simulink model "CONTROL_TESTING"  (R2024a)
settings: Solver=VariableStepAuto  StartTime=0.0  StopTime=inf  RelTol=1e-3
values from neighbouring files (symbols this model uses):
  C = 0    [CONTROL_TESTING_VARIABLES.m]
  Direction_Pin = 0    [CONTROL_TESTING_VARIABLES.m]
  EN_Pin = 1    [CONTROL_TESTING_VARIABLES.m]
  FP_New_Max_Angle = 360    [CONTROL_TESTING_VARIABLES.m]
  FP_New_Max_Percent = 255    [CONTROL_TESTING_VARIABLES.m]
  FP_New_Min_Angle = 0    [CONTROL_TESTING_VARIABLES.m]
  FP_New_Min_Percent = 0    [CONTROL_TESTING_VARIABLES.m]
  FP_Old_Max = 5    [CONTROL_TESTING_VARIABLES.m]
  FP_Old_Min = 0    [CONTROL_TESTING_VARIABLES.m]
  TB_New_Max_Angle = 360    [CONTROL_TESTING_VARIABLES.m]
  TB_New_Max_Percent = 255    [CONTROL_TESTING_VARIABLES.m]
  TB_New_Min_Angle = 0    [CONTROL_TESTING_VARIABLES.m]
  TB_New_Min_Percent = 0    [CONTROL_TESTING_VARIABLES.m]
  TB_Old_Max = 5    [CONTROL_TESTING_VARIABLES.m]
  TB_Old_Min = 0    [CONTROL_TESTING_VARIABLES.m]
libraries: fl_lib x11, nesl_utility x9, arduinolib x4, ee_lib x3, sdl_lib x1
(part 2 of 2)

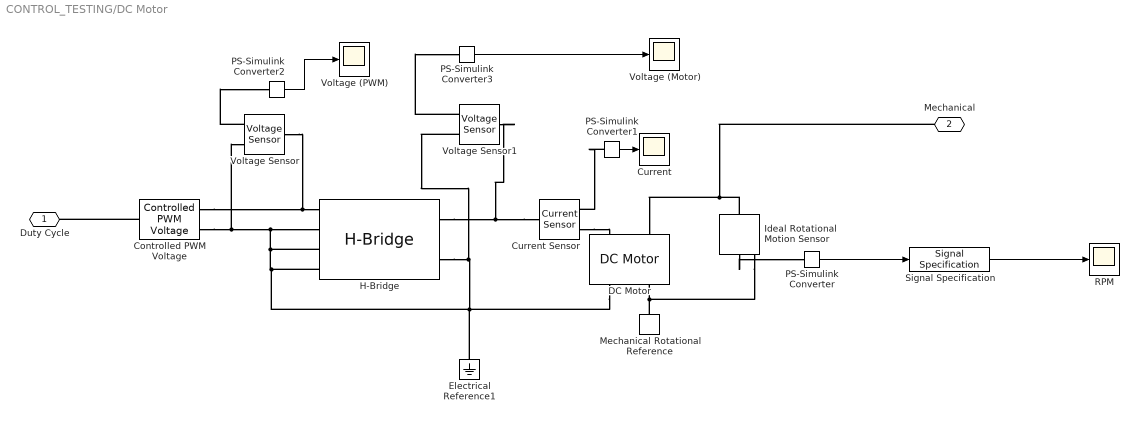
== system CONTROL_TESTING/DC Motor ==
  Controlled PWM Voltage : ee_lib/Integrated Circuits/Controlled PWM Voltage  F=2000 Hz  TD=0 s  pulse_width_offset=0 s  pulse_min=0 s  pwm_or_av=ee.enum.pwm_or_av.averaged  event_type=1  sample_time=1e-6 s  Vmin=0 V  Vmax=5 V  Vm=5 V  u_min=0  u_max=255
      settings: InternalSimscapePortConfiguration="{\"Bottom\":[],\"Left\":[{\"id\":\"u\",\"label\":\"u\",\"type\":\"input\"}],\"Right\":[{\"id\":\"p2\",\"label\":\"PWM\",\"type\":\"foundation.electrical.electrical\"},{\"id\":\"n2\",\"label\":\"REF\",\"type\":\"foundation.electrical.electrical\"}],\"Top\":[]}"
  Current : Scope
  Current Sensor : fl_lib/Electrical/Electrical Sensors/Current Sensor
  DC Motor : ee_lib/Electromechanical/Brushed Motors/DC Motor  field_option=ee.enum.field_option.pm  Rf=100 Ohm  Lf=1 H  Laf=0.15 H  If0=0 A  parameterization=ee.enum.dcparam_option.load_speed  Ra=3.9 Ohm  La=0.01 H  emf_or_torque=ee.enum.emf_or_torque.kv  Kv=0.072e-3 V/rpm  Ki=6.876e-4 N*m/A  T_stall=0.24e-3 N*m  w_max=4000 rpm  w_rated=2500 rpm  P_rated=10 W  V_rated=12 V  lam_param=ee.enum.lam_param.damping  i_noload=0 A  V_i_noload=1.5 V  J=0.0002 kg*m^2  lam=0.5e-5 N*m/(rad/s)  speed0=0 rpm  enable_fault_armature=simscape.enum.onoff.off  rev_faulted=1 / 3  G_faulted_armature=1e-5 S  fault_trigger_armature=ee.enum.faults.faultTrigger.temporal  t_fault_armature=1 s  max_permissible_current_armature=inf A  t_fail_on_current_armature=1 s  enable_fault_field=simscape.enum.onoff.off  G_faulted_field=1e-5 S  fault_trigger_field=ee.enum.faults.faultTrigger.temporal  t_fault_field=1 s  max_permissible_current_field=inf A  t_fail_on_current_field=1 s  fault_action=simscape.enum.assert.action.none  alpha=3.93e-3 1/K  Tmeas=25 degC  thermal_mass=100 J/K  initial_temperature=25 degC
      settings: LogSimulationData=on
  Electrical Reference1 : fl_lib/Electrical/Electrical Elements/Electrical Reference
  H-Bridge : ee_lib/Semiconductors & Converters/Converters/H-Bridge  supply_ports=ee.enum.supply_ports.hidesupply  pwm_or_av=ee.enum.pwm_or_av.averaged  regenerative_braking_mode=ee.enum.converters.regenerative_braking_mode.depends_on_rev  discontinuous=ee.enum.current_profile.continuous  freewheeling_mode=ee.enum.converters.freewheeling_mode.one_switch_one_diode  Rload=10 Ohm  Lload=1e-5 H  F=10 kHz  Venable=0.1 V  Vmax=5 V  Vreverse=2.5 V  Vbrake=0.1 V  Vm=12 V  Ron=0.1 Ohm  Don=0.05 Ohm  Goff=1e-6 S  Tmeas=298.15 K  Ron2=0.1 Ohm  Don2=0.05 Ohm  Tmeas2=398.15 K  thermal_mass=100 J/K  initial_temperature=298.15 K
  Ideal Rotational Motion Sensor : fl_lib/Mechanical/Mechanical Sensors/Ideal Rotational Motion Sensor  reference=foundation.enum.MeasurementReference.difference  acceleration_port=false  velocity_port=true  position_port=true  wrap_angle=simscape.enum.onoff.off  offset=0 rad
  Mechanical Rotational Reference : fl_lib/Mechanical/Rotational Elements/Mechanical Rotational Reference
  PS-Simulink Converter{,1..3} (4 alike) : nesl_utility/PS-Simulink Converter  PhysicalDomain=network_engine_domain  SubClassName=ps_output  LeftPortType=input  RightPortType=output  PseudoPeriodic=off  Frequencies=[]  VectorFormat=inherit  Unit=inherit  AffineConversion=off
  RPM : Scope
  Signal Specification : SignalSpecification  Unit=rpm
  Voltage (Motor) : Scope
  Voltage (PWM) : Scope
      settings: Priority=3
  Voltage Sensor : fl_lib/Electrical/Electrical Sensors/Voltage Sensor
  Voltage Sensor1 : fl_lib/Electrical/Electrical Sensors/Voltage Sensor
  Duty Cycle : PMIOPort  Side=Left
  Mechanical : PMIOPort  Port=2  Side=Right
  wires:
  PS-Simulink Converter1/1 -> Current/1
  PS-Simulink Converter/1 -> Signal Specification/1
  PS-Simulink Converter3/1 -> Voltage (Motor)/1
  PS-Simulink Converter2/1 -> Voltage (PWM)/1
  Signal Specification/1 -> RPM/1
  connections:
  H-Bridge/LConn4 -- Electrical Reference1/LConn1 -- Voltage Sensor1/RConn2 -- H-Bridge/RConn2 -- DC Motor/RConn1 -- H-Bridge/LConn3 -- Controlled PWM Voltage/RConn2 -- Voltage Sensor/RConn2 -- H-Bridge/LConn2
  H-Bridge/LConn1 -- Controlled PWM Voltage/RConn1 -- Voltage Sensor/LConn1
  PS-Simulink Converter1/LConn1 -- Current Sensor/RConn1
  Ideal Rotational Motion Sensor/LConn1 -- Mechanical/RConn1 -- DC Motor/LConn2
  Current Sensor/LConn1 -- Voltage Sensor1/LConn1 -- H-Bridge/RConn1
  Voltage Sensor1/RConn1 -- PS-Simulink Converter3/LConn1
  Ideal Rotational Motion Sensor/RConn1 -- Mechanical Rotational Reference/LConn1 -- DC Motor/RConn2
  Current Sensor/RConn2 -- DC Motor/LConn1
  Voltage Sensor/RConn1 -- PS-Simulink Converter2/LConn1
  Ideal Rotational Motion Sensor/RConn2 -- PS-Simulink Converter/LConn1
  Controlled PWM Voltage/LConn1 -- Duty Cycle/RConn1

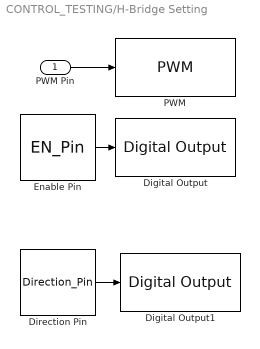
== system CONTROL_TESTING/H-Bridge Setting ==
  PWM Pin : Inport
  Digital Output : arduinolib/Digital Output  pinNumber=9  Direction=output  blockPlatform=arduino
  Digital Output1 : arduinolib/Digital Output  pinNumber=10  Direction=output  blockPlatform=arduino
  Direction Pin : Constant  Value=Direction_Pin
  Enable Pin : Constant  Value=EN_Pin
  PWM : arduinolib/PWM  pinNumber=5  frequencyType=Default  desiredFrequency=490.2  achievableFrequency=490.2
  wires:
  PWM Pin/1 -> PWM/1
  Enable Pin/1 -> Digital Output/1
  Direction Pin/1 -> Digital Output1/1

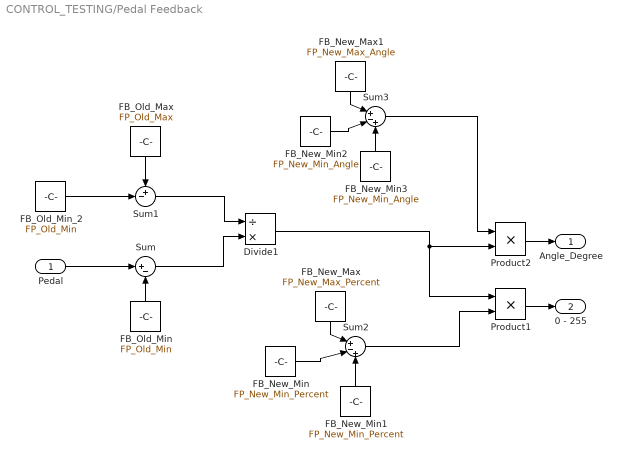
== system CONTROL_TESTING/Pedal Feedback ==
  Pedal : Inport
  Divide1 : Product  Inputs=/*
  FB_New_Max : Constant  Value=FP_New_Max_Percent
  FB_New_Max1 : Constant  Value=FP_New_Max_Angle
  FB_New_Min : Constant  Value=FP_New_Min_Percent
  FB_New_Min1 : Constant  Value=FP_New_Min_Percent
  FB_New_Min2 : Constant  Value=FP_New_Min_Angle
  FB_New_Min3 : Constant  Value=FP_New_Min_Angle
  FB_Old_Max : Constant  Value=FP_Old_Max
  FB_Old_Min : Constant  Value=FP_Old_Min
  FB_Old_Min_2 : Constant  Value=FP_Old_Min
  Product1 : Product
  Product2 : Product
  Sum : Sum  Inputs=|+-
  Sum1 : Sum  Inputs=+-|
  Sum2 : Sum  Inputs=|+-+
  Sum3 : Sum  Inputs=|+-+
  Angle_Degree : Outport
  0 - 255 : Outport  Port=2
  wires:
  FB_New_Min1/1 -> Sum2/3
  Product1/1 -> 0 - 255/1
  Divide1/1 -> Product1/1, Product2/2
  Sum2/1 -> Product1/2
  FB_New_Min2/1 -> Sum3/2
  FB_New_Max1/1 -> Sum3/1
  FB_New_Min/1 -> Sum2/2
  Sum3/1 -> Product2/1
  Sum/1 -> Divide1/2
  FB_Old_Min/1 -> Sum/2
  FB_New_Min3/1 -> Sum3/3
  FB_New_Max/1 -> Sum2/1
  FB_Old_Min_2/1 -> Sum1/2
  Sum1/1 -> Divide1/1
  Product2/1 -> Angle_Degree/1
  FB_Old_Max/1 -> Sum1/1
  Pedal/1 -> Sum/1

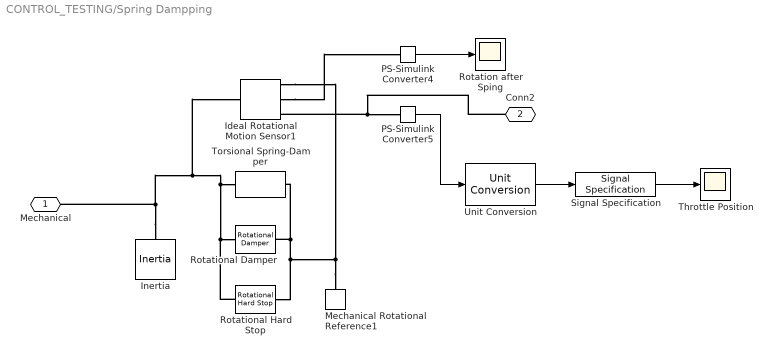
== system CONTROL_TESTING/Spring Dampping ==
  Ideal Rotational Motion Sensor1 : fl_lib/Mechanical/Mechanical Sensors/Ideal Rotational Motion Sensor  reference=foundation.enum.MeasurementReference.difference  acceleration_port=false  velocity_port=true  position_port=true  wrap_angle=true  offset=0 deg
  Inertia : fl_lib/Mechanical/Rotational Elements/Inertia  inertia=0.00000000001 kg*m^2  num_ports=foundation.enum.numPorts2.one  w_specify=off  w_priority=High  w=0 rad/s  w_nominal_specify=off  w_nominal_value=1  w_nominal_unit=rad/s  t_specify=off  t_priority=None  t=0 N*m  t_nominal_specify=off  t_nominal_value=1  t_nominal_unit=N*m
  Mechanical Rotational Reference1 : fl_lib/Mechanical/Rotational Elements/Mechanical Rotational Reference
  PS-Simulink Converter4 : nesl_utility/PS-Simulink Converter  PhysicalDomain=network_engine_domain  SubClassName=ps_output  LeftPortType=input  RightPortType=output  PseudoPeriodic=off  Frequencies=[]  VectorFormat=inherit  Unit=inherit  AffineConversion=off
  PS-Simulink Converter5 : nesl_utility/PS-Simulink Converter  PhysicalDomain=network_engine_domain  SubClassName=ps_output  LeftPortType=input  RightPortType=output  PseudoPeriodic=off  Frequencies=[]  VectorFormat=inherit  Unit=inherit  AffineConversion=off
  Rotation after Sping : Scope
  Rotational Damper : fl_lib/Mechanical/Rotational Elements/Rotational Damper  D=0.00001 N*m*s/rad  w_specify=off  w_priority=None  w=0 rad/s  w_nominal_specify=off  w_nominal_value=1  w_nominal_unit=rad/s  t_specify=off  t_priority=None  t=0 N*m  t_nominal_specify=off  t_nominal_value=1  t_nominal_unit=N*m
  Rotational Hard Stop : fl_lib/Mechanical/Rotational Elements/Rotational Hard Stop  upper_bnd=27.73873597 rad  lower_bnd=0 rad  model=simscape.enum.hardstop.smooth  stiff_up=1e6 N*m/rad  stiff_low=1e6 N*m/rad  D_up=0.1 N*m*s/rad  D_low=0.1 N*m*s/rad  transition=0.001 rad  coeff_rest=0.7  w_tol=0.1 rad/s  trq_tol=0.001 N*m  w_specify=off  w_priority=None  w=0 rad/s  w_nominal_specify=off  w_nominal_value=1  w_nominal_unit=rad/s  t_specify=off  t_priority=None  t=0 N*m  t_nominal_specify=off  t_nominal_value=1  t_nominal_unit=N*m  phi_specify=off  phi_priority=High  phi=0 rad  phi_nominal_specify=off  phi_nominal_value=1  phi_nominal_unit=rad  M_specify=off  M_priority=None  M=0
  Signal Specification : SignalSpecification  Unit=deg
  Throttle Position : Scope
  Torsional Spring-Damper : sdl_lib/Couplings & Drives/Torsional Spring-Damper  k=0.0020928 N*m/rad  mu_visc=0 N*m*s/rad  trq_coulomb=0 N*m  static_kinetic_ratio=10  w_tol=0.001 rad/s  model_hardstop=sdl.enum.hardStopOffOn.off  upper_bound=10 deg  lower_bound=-10 deg  hardstop_model=simscape.enum.hardstop.smooth  k_endstop=1e6 N*m/rad  D_endstop=10 N*m*s/rad  transition=0.001 rad  coeff_rest=0.7  w_tol_hardstop=0.1 rad/s  trq_tol=0.001 N*m  x0=0 deg
      settings: InternalSimscapePortConfiguration="{\"Bottom\":[],\"Left\":[{\"id\":\"R\",\"label\":\"R\",\"type\":\"foundation.mechanical.rotational.rotational\"}],\"Right\":[{\"id\":\"C\",\"label\":\"C\",\"type\":\"foundation.mechanical.rotational.rotational\"}],\"Top\":[]}"
  Unit Conversion : UnitConversion
  Mechanical : PMIOPort  Side=Left
  Conn2 : PMIOPort  Port=2  Side=Right
  wires:
  PS-Simulink Converter4/1 -> Rotation after Sping/1
  Signal Specification/1 -> Throttle Position/1
  PS-Simulink Converter5/1 -> Unit Conversion/1
  Unit Conversion/1 -> Signal Specification/1
  connections:
  Ideal Rotational Motion Sensor1/RConn2 -- PS-Simulink Converter4/LConn1
  Conn2/RConn1 -- Ideal Rotational Motion Sensor1/RConn3 -- PS-Simulink Converter5/LConn1
  Inertia/LConn1 -- Ideal Rotational Motion Sensor1/LConn1 -- Torsional Spring-Damper/LConn1 -- Rotational Hard Stop/LConn1 -- Rotational Damper/LConn1 -- Mechanical/RConn1
  Mechanical Rotational Reference1/LConn1 -- Rotational Hard Stop/RConn1 -- Torsional Spring-Damper/RConn1 -- Rotational Damper/RConn1 -- Ideal Rotational Motion Sensor1/RConn1

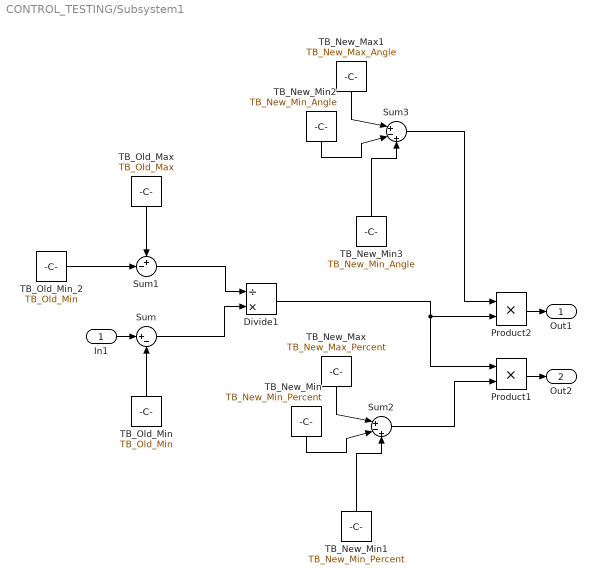
== system CONTROL_TESTING/Subsystem1 ==
  In1 : Inport
  Divide1 : Product  Inputs=/*
  Product1 : Product
  Product2 : Product
  Sum : Sum  Inputs=|+-
  Sum1 : Sum  Inputs=+-|
  Sum2 : Sum  Inputs=|+-+
  Sum3 : Sum  Inputs=|+-+
  TB_New_Max : Constant  Value=TB_New_Max_Percent
  TB_New_Max1 : Constant  Value=TB_New_Max_Angle
  TB_New_Min : Constant  Value=TB_New_Min_Percent
  TB_New_Min1 : Constant  Value=TB_New_Min_Percent
  TB_New_Min2 : Constant  Value=TB_New_Min_Angle
  TB_New_Min3 : Constant  Value=TB_New_Min_Angle
  TB_Old_Max : Constant  Value=TB_Old_Max
  TB_Old_Min : Constant  Value=TB_Old_Min
  TB_Old_Min_2 : Constant  Value=TB_Old_Min
  Out1 : Outport
  Out2 : Outport  Port=2
  wires:
  Sum1/1 -> Divide1/1
  Divide1/1 -> Product1/1, Product2/2
  Sum/1 -> Divide1/2
  Product2/1 -> Out1/1
  Product1/1 -> Out2/1
  TB_New_Max/1 -> Sum2/1
  Sum2/1 -> Product1/2
  TB_New_Min3/1 -> Sum3/3
  TB_Old_Max/1 -> Sum1/1
  TB_New_Min1/1 -> Sum2/3
  Sum3/1 -> Product2/1
  TB_Old_Min/1 -> Sum/2
  TB_New_Min2/1 -> Sum3/2
  TB_New_Max1/1 -> Sum3/1
  TB_New_Min/1 -> Sum2/2
  TB_Old_Min_2/1 -> Sum1/2
  In1/1 -> Sum/1
